simulink model "lowfilter"  (R2020a)
settings: Solver=VariableStepAuto  StartTime=0.0  StopTime=550/20  RelTol=1e-3
libraries: dspsrcs4 x1
settings Model: Creator=User  LastModifiedBy=User

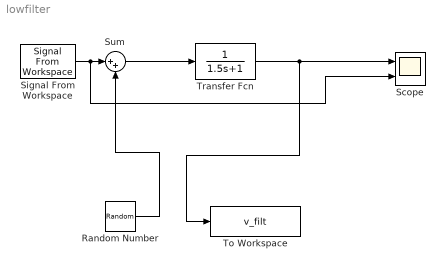
== system lowfilter ==
  Random Number : RandomNumber  Variance=0.1  SampleTime=0.1
  Scope : Scope  NumInputPorts=2
  Signal From Workspace : dspsrcs4/Signal From Workspace  X=v  Ts=0.05  nsamps=1  OutputAfterFinalValue=Setting to zero  ignoreOrWarnInputAndFrameLengths=off  OutputFrames=off
  Sum : Sum  Inputs=|++
  To Workspace : ToWorkspace  VariableName=v_filt  SampleTime=-1
  Transfer Fcn : TransferFcn  Denominator=[1.5 1]
  wires:
  Transfer Fcn/1 -> To Workspace/1, Scope/1
  Signal From Workspace/1 -> Scope/2, Sum/1
  Random Number/1 -> Sum/2
  Sum/1 -> Transfer Fcn/1
